simulink model "LQG_controller"  (R2024b)
settings: Solver=VariableStepAuto  StartTime=0.0  StopTime=100  RelTol=1e-3
values from neighbouring files (symbols this model uses):
  A = [0 , 1, 0, 0, 0, 0 ... (first row only)    [part_E.m]    (also in part_F.m; part_G.m; part_c.m; part_d.m)
  B = [0 ... (first row only)    [part_F.m]    (also in part_G.m; part_c.m; part_d.m)
  C_all = [1, 0, 0, 0, 0, 0 ... (first row only)    [part_G.m]
  C_obs = [1, 0, 0, 0, 0, 0;]    [part_G.m]
  D_all = [0; 0; 0; 0; 0; 0]    [part_G.m]
  D_obs = [0]    [part_G.m]
  N = 0    [part_G.m]
  Q = 0.1    [part_G.m]    (also in part_d.m = [1, 0, 0, 0, 0, 0)
  R = 0.0001    [part_G.m]    (also in part_d.m = [0.00001])
  x0 = [1; 0; pi/2; 0; -pi/10; 0;]    [part_F.m]    (also in part_G.m; part_d.m)
  x_hat0 = [0; 0; 0; 0; 0; 0;]    [part_G.m]
undefined symbols (not defined in the file or in its folder): Continuous, K, Time
libraries: ctrlSharedLib x1
settings Model: Creator=timsweeney  LastModifiedBy=timsweeney

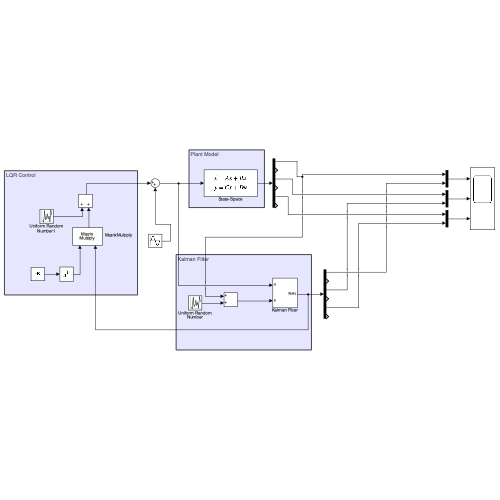
[thumbnail: Simulink's stored preview of the top-level diagram]
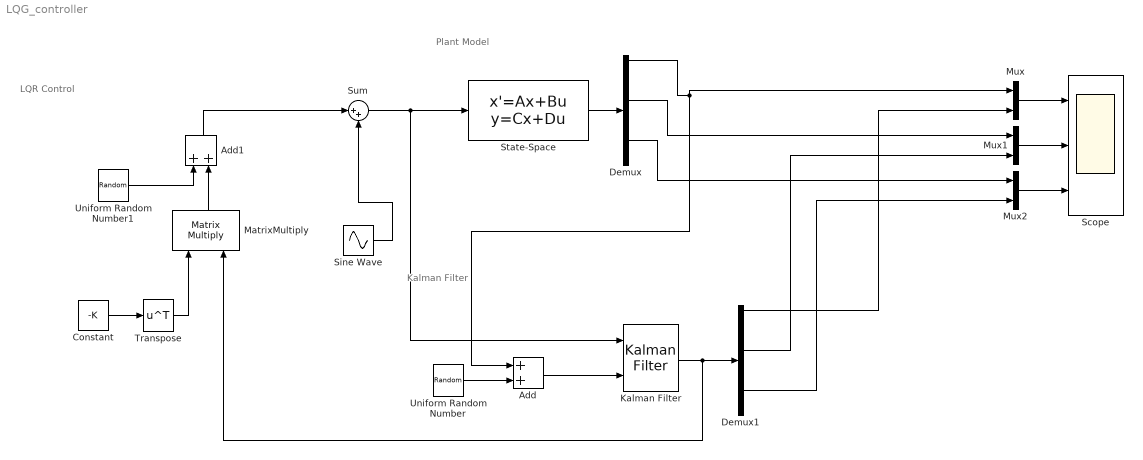
== system LQG_controller ==
  note: Kalman Filter
  note: Plant Model
  note: LQR Control
  Add : Sum
  Add1 : Sum
  Constant : Constant  Value=-K
  Demux : Demux  Outputs=6
  Demux1 : Demux  Outputs=6
  Kalman Filter : ctrlSharedLib/Kalman Filter  TimeDomain=Continuous-Time  UseCurrentEstimator=on  ModelSource=Individual A, B, C, D matrices  ModelSourceVariable=ss(0.95,1,1,0,1)  A=A  B=B  C=C_obs  D=D_obs  NumberOfStates=6  NumberOfInputs=1  NumberOfOutputs=6  InitialEstimateSource=Dialog  X0=x_hat0  P0=10  UseK=off  UseGH=off  NumberOfProcessNoiseInputs=1  G=1  TimeInvariantG=on  H=0  TimeInvariantH=on  Q=Q  TimeInvariantQ=on  R=R  TimeInvariantR=on  N=N  TimeInvariantN=on  AddInputPort=on  AddEnablePort=off  OutputEstimatedY=off  OutputP=off  Ts=-1
  MatrixMultiply : Product  Multiplication=Matrix(*)
  Mux : Mux  Inputs=2
  Mux1 : Mux  Inputs=2
  Mux2 : Mux  Inputs=2
  Scope : Scope  NumInputPorts=3
  Sine Wave : Sin  SampleTime=0
  State-Space : StateSpace  A=A  B=B  C=C_all  D=D_all  InitialCondition=x0
  Sum : Sum  Inputs=|++
  Transpose : Math  Operator=transpose
  Uniform Random Number : UniformRandomNumber  Minimum=-Q  Maximum=Q
  Uniform Random Number1 : UniformRandomNumber  Minimum=-10  Maximum=10
  wires:
  State-Space/1 -> Demux/1
  Demux1/1 -> Mux/2
  Demux/3 -> Mux1/1
  Demux1/3 -> Mux1/2
  Demux/5 -> Mux2/1
  Mux2/1 -> Scope/3
  Mux1/1 -> Scope/2
  Mux/1 -> Scope/1
  Demux1/5 -> Mux2/2
  Uniform Random Number/1 -> Add/2
  Add/1 -> Kalman Filter/2
  Kalman Filter/1 -> MatrixMultiply/2, Demux1/1
  Constant/1 -> Transpose/1
  Transpose/1 -> MatrixMultiply/1
  MatrixMultiply/1 -> Add1/2
  Uniform Random Number1/1 -> Add1/1
  Add1/1 -> Sum/1
  Demux/1 -> Add/1, Mux/1
  Sum/1 -> State-Space/1, Kalman Filter/1
  Sine Wave/1 -> Sum/2
